simulink model "Q54"  (R2023a)
settings: Solver=VariableStepAuto  StartTime=0.0  StopTime=10.0  MaxStep=0.001  RelTol=1e-3
settings Model: Creator=Physics Library  LastModifiedBy=Physics Library

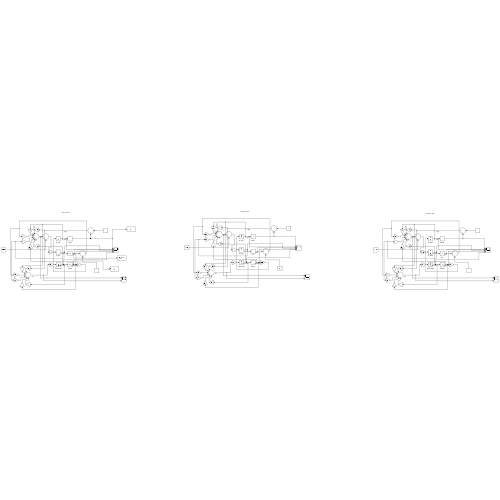
[thumbnail: Simulink's stored preview of the top-level diagram]
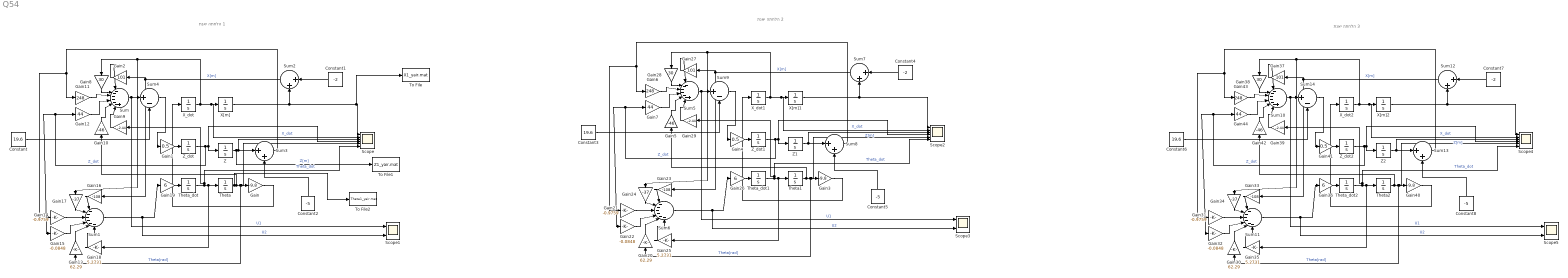
== system Q54 ==
  note: תנאי התחלה 1
  note: תנאי התחלה 2
  note: תנאי התחלה 3
  Constant : Constant  Value=19.6
  Constant1 : Constant  Value=-2
  Constant2 : Constant  Value=-5
  Constant3 : Constant  Value=19.6
  Constant4 : Constant  Value=-2
  Constant5 : Constant  Value=-5
  Constant6 : Constant  Value=19.6
  Constant7 : Constant  Value=-2
  Constant8 : Constant  Value=-5
  Gain : Gain  Gain=-9.8
  Gain1 : Gain  Gain=0.5
  Gain10 : Gain  Gain=-46
  Gain11 : Gain  Gain=248
  Gain12 : Gain  Gain=44
  Gain13 : Gain  Gain=62.29
  Gain14 : Gain  Gain=-0.9759
  Gain15 : Gain  Gain=-0.0848
  Gain16 : Gain  Gain=-108
  Gain17 : Gain  Gain=-37
  Gain18 : Gain  Gain=5.2731
  Gain19 : Gain  Gain=6
  Gain2 : Gain  Gain=101
  Gain20 : Gain  Gain=62.29
  Gain21 : Gain  Gain=-0.9759
  Gain22 : Gain  Gain=-0.0848
  Gain23 : Gain  Gain=-108
  Gain24 : Gain  Gain=-37
  Gain25 : Gain  Gain=5.2731
  Gain26 : Gain  Gain=6
  Gain27 : Gain  Gain=101
  Gain28 : Gain  Gain=30
  Gain29 : Gain  Gain=-2.44
  Gain3 : Gain  Gain=-9.8
  Gain30 : Gain  Gain=62.29
  Gain31 : Gain  Gain=-0.9759
  Gain32 : Gain  Gain=-0.0848
  Gain33 : Gain  Gain=-108
  Gain34 : Gain  Gain=-37
  Gain35 : Gain  Gain=5.2731
  Gain36 : Gain  Gain=6
  Gain37 : Gain  Gain=101
  Gain38 : Gain  Gain=30
  Gain39 : Gain  Gain=-2.44
  Gain4 : Gain  Gain=0.5
  Gain40 : Gain  Gain=-9.8
  Gain41 : Gain  Gain=0.5
  Gain42 : Gain  Gain=-46
  Gain43 : Gain  Gain=248
  Gain44 : Gain  Gain=44
  Gain5 : Gain  Gain=-46
  Gain6 : Gain  Gain=248
  Gain7 : Gain  Gain=44
  Gain8 : Gain  Gain=30
  Gain9 : Gain  Gain=-2.44
  Scope : Scope  NumInputPorts=6
  Scope1 : Scope  NumInputPorts=2
  Scope2 : Scope  NumInputPorts=6
  Scope3 : Scope  NumInputPorts=2
  Scope4 : Scope  NumInputPorts=6
  Scope5 : Scope  NumInputPorts=2
  Sum : Sum  Inputs=|------+
  Sum1 : Sum  Inputs=|------
  Sum10 : Sum  Inputs=|------+
  Sum11 : Sum  Inputs=|------
  Sum{2..3,7..8,12..13} (6 alike) : Sum  Inputs=|++
  Sum14 : Sum  Inputs=|+-
  Sum4 : Sum  Inputs=|+-
  Sum5 : Sum  Inputs=|------+
  Sum6 : Sum  Inputs=|------
  Sum9 : Sum  Inputs=|+-
  Theta : Integrator  InitialCondition=pi/6
  Theta1 : Integrator  InitialCondition=pi/3
  Theta2 : Integrator  InitialCondition=pi/8
  Theta_dot : Integrator
  Theta_dot1 : Integrator  InitialCondition=10
  Theta_dot2 : Integrator
  To File : ToFile  Filename=X1_yair.mat  SaveFormat=Timeseries
  To File1 : ToFile  Filename=Z1_yair.mat  SaveFormat=Timeseries
  To File2 : ToFile  Filename=Theta1_yair.mat  SaveFormat=Timeseries
  X[m] : Integrator
  X[m]1 : Integrator  InitialCondition=5
  X[m]2 : Integrator  InitialCondition=5
  X_dot : Integrator
  X_dot1 : Integrator
  X_dot2 : Integrator  InitialCondition=1
  Z : Integrator  InitialCondition=1
  Z1 : Integrator  InitialCondition=1
  Z2 : Integrator  InitialCondition=10
  Z_dot : Integrator
  Z_dot1 : Integrator  InitialCondition=1
  Z_dot2 : Integrator  InitialCondition=-1
  wires:
  Gain/1 -> X_dot/1
  Sum2/1 -> Gain2/1, Gain16/1  "X[m]"
  X_dot/1 -> Gain17/1, Gain8/1, X[m]/1, Scope/2  "X_dot"
  Sum3/1 -> Gain14/1, Gain11/1
  Z_dot/1 -> Gain12/1, Gain15/1, Scope/4, Z/1  "Z_dot"
  Theta/1 -> To File2/1, Gain10/1, Scope/5, Gain/1, Gain13/1  "Theta[rad]"
  Theta_dot/1 -> Gain18/1, Theta/1, Gain9/1, Scope/6  "Theta_dot"
  Gain2/1 -> Sum/1
  Gain8/1 -> Sum/2
  Gain9/1 -> Sum/6
  Gain10/1 -> Sum/5
  Gain11/1 -> Sum/3
  Gain12/1 -> Sum/4
  Gain1/1 -> Z_dot/1
  Sum4/1 -> Gain1/1
  Gain15/1 -> Sum1/4
  Gain17/1 -> Sum1/2
  Gain18/1 -> Sum1/6
  Gain13/1 -> Sum1/5
  Sum1/1 -> Scope1/2, Gain19/1  "U2"
  Gain14/1 -> Sum1/3
  Gain16/1 -> Sum1/1
  Gain19/1 -> Theta_dot/1
  X[m]/1 -> To File/1, Scope/1, Sum2/2
  Constant1/1 -> Sum2/1
  Z/1 -> To File1/1, Scope/3, Sum3/1  "Z[m]"
  Constant2/1 -> Sum3/2
  Sum/1 -> Scope1/1, Sum4/1  "U1"
  Constant/1 -> Sum4/2
  Constant3/1 -> Sum9/2
  Gain3/1 -> X_dot1/1
  Gain23/1 -> Sum6/1
  Z1/1 -> Scope2/3, Sum8/1  "Z[m]"
  Sum6/1 -> Scope3/2, Gain26/1  "U2"
  Constant5/1 -> Sum8/2
  Sum9/1 -> Gain4/1
  Gain20/1 -> Sum6/5
  Gain28/1 -> Sum5/2
  Gain29/1 -> Sum5/6
  Z_dot1/1 -> Gain7/1, Gain22/1, Scope2/4, Z1/1  "Z_dot"
  Sum8/1 -> Gain21/1, Gain6/1
  Gain4/1 -> Z_dot1/1
  Sum7/1 -> Gain27/1, Gain23/1  "X[m]"
  Gain7/1 -> Sum5/4
  Gain24/1 -> Sum6/2
  Gain25/1 -> Sum6/6
  Gain5/1 -> Sum5/5
  Gain22/1 -> Sum6/4
  Gain21/1 -> Sum6/3
  X[m]1/1 -> Scope2/1, Sum7/2
  Theta_dot1/1 -> Gain25/1, Theta1/1, Gain29/1, Scope2/6  "Theta_dot"
  Theta1/1 -> Gain5/1, Scope2/5, Gain3/1, Gain20/1  "Theta[rad]"
  Gain6/1 -> Sum5/3
  X_dot1/1 -> Gain24/1, Gain28/1, X[m]1/1, Scope2/2  "X_dot"
  Sum5/1 -> Scope3/1, Sum9/1  "U1"
  Gain27/1 -> Sum5/1
  Gain26/1 -> Theta_dot1/1
  Constant4/1 -> Sum7/1
  Gain37/1 -> Sum10/1
  Gain43/1 -> Sum10/3
  X[m]2/1 -> Scope4/1, Sum12/2
  Gain42/1 -> Sum10/5
  Theta_dot2/1 -> Gain35/1, Theta2/1, Gain39/1, Scope4/6  "Theta_dot"
  X_dot2/1 -> Gain34/1, Gain38/1, X[m]2/1, Scope4/2  "X_dot"
  Sum13/1 -> Gain31/1, Gain43/1
  Gain31/1 -> Sum11/3
  Z_dot2/1 -> Gain44/1, Gain32/1, Scope4/4, Z2/1  "Z_dot"
  Sum12/1 -> Gain37/1, Gain33/1  "X[m]"
  Theta2/1 -> Gain42/1, Scope4/5, Gain40/1, Gain30/1  "Theta[rad]"
  Gain35/1 -> Sum11/6
  Gain44/1 -> Sum10/4
  Gain39/1 -> Sum10/6
  Gain38/1 -> Sum10/2
  Gain30/1 -> Sum11/5
  Sum14/1 -> Gain41/1
  Gain32/1 -> Sum11/4
  Sum11/1 -> Scope5/2, Gain36/1  "U2"
  Constant7/1 -> Sum12/1
  Z2/1 -> Scope4/3, Sum13/1  "Z[m]"
  Constant8/1 -> Sum13/2
  Sum10/1 -> Scope5/1, Sum14/1  "U1"
  Gain34/1 -> Sum11/2
  Gain33/1 -> Sum11/1
  Gain41/1 -> Z_dot2/1
  Gain36/1 -> Theta_dot2/1
  Constant6/1 -> Sum14/2
  Gain40/1 -> X_dot2/1
